simulink model "UZ_EnDat_be4_optimizing_ctrs"  (R2023b)
settings: Solver=FixedStepDiscrete  StartTime=0  StopTime=0.002  RelTol=1e-3
model workspace (MAT data in the model file):
  Select = 0
libraries: hdlsllib x755, simulink x20, simulink_extras x4
(part 5 of 9)

== system UZ_EnDat_be4_optimizing_ctrs/UZ_ENDAT/ManualSerialize/padder/nibblepadding15 ==
  in : Inport
  padding : Subsystem  Commented=through
  padding1 : Subsystem
  padding2 : Subsystem
  padding3 : Subsystem
  out : Outport
  wires:
  in/1 -> padding3/1(in)
  padding2/1(out) -> padding1/1(in)
  padding3/1(out) -> padding2/1(in)
  padding1/1(out) -> padding/1(in)
  padding/1(out) -> out/1

== system UZ_EnDat_be4_optimizing_ctrs/UZ_ENDAT/ManualSerialize/padder/nibblepadding16 ==
  in : Inport
  padding : Subsystem  Commented=through
  padding1 : Subsystem
  padding2 : Subsystem
  padding3 : Subsystem
  out : Outport
  wires:
  in/1 -> padding3/1(in)
  padding2/1(out) -> padding1/1(in)
  padding3/1(out) -> padding2/1(in)
  padding1/1(out) -> padding/1(in)
  padding/1(out) -> out/1

== system UZ_EnDat_be4_optimizing_ctrs/UZ_ENDAT/ManualSerialize/padder/nibblepadding17 ==
  in : Inport
  padding : Subsystem  Commented=through
  padding1 : Subsystem
  padding2 : Subsystem
  padding3 : Subsystem
  out : Outport
  wires:
  in/1 -> padding3/1(in)
  padding2/1(out) -> padding1/1(in)
  padding3/1(out) -> padding2/1(in)
  padding1/1(out) -> padding/1(in)
  padding/1(out) -> out/1

== system UZ_EnDat_be4_optimizing_ctrs/UZ_ENDAT/ManualSerialize/padder/nibblepadding18 ==
  in : Inport
  padding : Subsystem  Commented=through
  padding1 : Subsystem
  padding2 : Subsystem
  padding3 : Subsystem
  out : Outport
  wires:
  in/1 -> padding3/1(in)
  padding2/1(out) -> padding1/1(in)
  padding3/1(out) -> padding2/1(in)
  padding1/1(out) -> padding/1(in)
  padding/1(out) -> out/1

== system UZ_EnDat_be4_optimizing_ctrs/UZ_ENDAT/ManualSerialize/padder/nibblepadding19 ==
  in : Inport
  padding : Subsystem  Commented=through
  padding1 : Subsystem
  padding2 : Subsystem
  padding3 : Subsystem
  out : Outport
  wires:
  in/1 -> padding3/1(in)
  padding2/1(out) -> padding1/1(in)
  padding3/1(out) -> padding2/1(in)
  padding1/1(out) -> padding/1(in)
  padding/1(out) -> out/1

== system UZ_EnDat_be4_optimizing_ctrs/UZ_ENDAT/ManualSerialize/padder/nibblepadding2 ==
  in : Inport
  padding : Subsystem  Commented=through
  padding1 : Subsystem
  padding2 : Subsystem
  padding3 : Subsystem
  out : Outport
  wires:
  in/1 -> padding3/1(in)
  padding2/1(out) -> padding1/1(in)
  padding3/1(out) -> padding2/1(in)
  padding1/1(out) -> padding/1(in)
  padding/1(out) -> out/1

== system UZ_EnDat_be4_optimizing_ctrs/UZ_ENDAT/ManualSerialize/padder/nibblepadding20 ==
  in : Inport
  padding : Subsystem  Commented=through
  padding1 : Subsystem
  padding2 : Subsystem
  padding3 : Subsystem
  out : Outport
  wires:
  in/1 -> padding3/1(in)
  padding2/1(out) -> padding1/1(in)
  padding3/1(out) -> padding2/1(in)
  padding1/1(out) -> padding/1(in)
  padding/1(out) -> out/1

== system UZ_EnDat_be4_optimizing_ctrs/UZ_ENDAT/ManualSerialize/padder/nibblepadding21 ==
  in : Inport
  padding : Subsystem  Commented=through
  padding1 : Subsystem
  padding2 : Subsystem
  padding3 : Subsystem
  out : Outport
  wires:
  in/1 -> padding3/1(in)
  padding2/1(out) -> padding1/1(in)
  padding3/1(out) -> padding2/1(in)
  padding1/1(out) -> padding/1(in)
  padding/1(out) -> out/1

== system UZ_EnDat_be4_optimizing_ctrs/UZ_ENDAT/ManualSerialize/padder/nibblepadding22 ==
  in : Inport
  padding : Subsystem  Commented=through
  padding1 : Subsystem
  padding2 : Subsystem
  padding3 : Subsystem
  out : Outport
  wires:
  in/1 -> padding3/1(in)
  padding2/1(out) -> padding1/1(in)
  padding3/1(out) -> padding2/1(in)
  padding1/1(out) -> padding/1(in)
  padding/1(out) -> out/1

== system UZ_EnDat_be4_optimizing_ctrs/UZ_ENDAT/ManualSerialize/padder/nibblepadding23 ==
  in : Inport
  padding : Subsystem  Commented=through
  padding1 : Subsystem
  padding2 : Subsystem
  padding3 : Subsystem
  out : Outport
  wires:
  in/1 -> padding3/1(in)
  padding2/1(out) -> padding1/1(in)
  padding3/1(out) -> padding2/1(in)
  padding1/1(out) -> padding/1(in)
  padding/1(out) -> out/1

== system UZ_EnDat_be4_optimizing_ctrs/UZ_ENDAT/ManualSerialize/padder/nibblepadding24 ==
  in : Inport
  padding : Subsystem  Commented=through
  padding1 : Subsystem
  padding2 : Subsystem
  padding3 : Subsystem
  out : Outport
  wires:
  in/1 -> padding3/1(in)
  padding2/1(out) -> padding1/1(in)
  padding3/1(out) -> padding2/1(in)
  padding1/1(out) -> padding/1(in)
  padding/1(out) -> out/1

== system UZ_EnDat_be4_optimizing_ctrs/UZ_ENDAT/ManualSerialize/padder/nibblepadding25 ==
  in : Inport
  padding : Subsystem  Commented=through
  padding1 : Subsystem
  padding2 : Subsystem
  padding3 : Subsystem
  out : Outport
  wires:
  in/1 -> padding3/1(in)
  padding2/1(out) -> padding1/1(in)
  padding3/1(out) -> padding2/1(in)
  padding1/1(out) -> padding/1(in)
  padding/1(out) -> out/1

== system UZ_EnDat_be4_optimizing_ctrs/UZ_ENDAT/ManualSerialize/padder/nibblepadding26 ==
  in : Inport
  padding : Subsystem  Commented=through
  padding1 : Subsystem
  padding2 : Subsystem
  padding3 : Subsystem
  out : Outport
  wires:
  in/1 -> padding3/1(in)
  padding2/1(out) -> padding1/1(in)
  padding3/1(out) -> padding2/1(in)
  padding1/1(out) -> padding/1(in)
  padding/1(out) -> out/1

== system UZ_EnDat_be4_optimizing_ctrs/UZ_ENDAT/ManualSerialize/padder/nibblepadding27 ==
  in : Inport
  padding : Subsystem  Commented=through
  padding1 : Subsystem
  padding2 : Subsystem
  padding3 : Subsystem
  out : Outport
  wires:
  in/1 -> padding3/1(in)
  padding2/1(out) -> padding1/1(in)
  padding3/1(out) -> padding2/1(in)
  padding1/1(out) -> padding/1(in)
  padding/1(out) -> out/1

== system UZ_EnDat_be4_optimizing_ctrs/UZ_ENDAT/ManualSerialize/padder/nibblepadding28 ==
  in : Inport
  padding : Subsystem  Commented=through
  padding1 : Subsystem
  padding2 : Subsystem
  padding3 : Subsystem
  out : Outport
  wires:
  in/1 -> padding3/1(in)
  padding2/1(out) -> padding1/1(in)
  padding3/1(out) -> padding2/1(in)
  padding1/1(out) -> padding/1(in)
  padding/1(out) -> out/1

== system UZ_EnDat_be4_optimizing_ctrs/UZ_ENDAT/ManualSerialize/padder/nibblepadding29 ==
  in : Inport
  padding : Subsystem  Commented=through
  padding1 : Subsystem
  padding2 : Subsystem
  padding3 : Subsystem
  out : Outport
  wires:
  in/1 -> padding3/1(in)
  padding2/1(out) -> padding1/1(in)
  padding3/1(out) -> padding2/1(in)
  padding1/1(out) -> padding/1(in)
  padding/1(out) -> out/1

== system UZ_EnDat_be4_optimizing_ctrs/UZ_ENDAT/ManualSerialize/padder/nibblepadding3 ==
  in : Inport
  padding : Subsystem  Commented=through
  padding1 : Subsystem
  padding2 : Subsystem
  padding3 : Subsystem
  out : Outport
  wires:
  in/1 -> padding3/1(in)
  padding2/1(out) -> padding1/1(in)
  padding3/1(out) -> padding2/1(in)
  padding1/1(out) -> padding/1(in)
  padding/1(out) -> out/1

== system UZ_EnDat_be4_optimizing_ctrs/UZ_ENDAT/ManualSerialize/padder/nibblepadding30 ==
  in : Inport
  padding : Subsystem  Commented=through
  padding1 : Subsystem
  padding2 : Subsystem
  padding3 : Subsystem
  out : Outport
  wires:
  in/1 -> padding3/1(in)
  padding2/1(out) -> padding1/1(in)
  padding3/1(out) -> padding2/1(in)
  padding1/1(out) -> padding/1(in)
  padding/1(out) -> out/1

== system UZ_EnDat_be4_optimizing_ctrs/UZ_ENDAT/ManualSerialize/padder/nibblepadding4 ==
  in : Inport
  padding : Subsystem  Commented=through
  padding1 : Subsystem
  padding2 : Subsystem
  padding3 : Subsystem
  out : Outport
  wires:
  in/1 -> padding3/1(in)
  padding2/1(out) -> padding1/1(in)
  padding3/1(out) -> padding2/1(in)
  padding1/1(out) -> padding/1(in)
  padding/1(out) -> out/1

== system UZ_EnDat_be4_optimizing_ctrs/UZ_ENDAT/ManualSerialize/padder/nibblepadding5 ==
  in : Inport
  padding : Subsystem  Commented=through
  padding1 : Subsystem
  padding2 : Subsystem
  padding3 : Subsystem
  out : Outport
  wires:
  in/1 -> padding3/1(in)
  padding2/1(out) -> padding1/1(in)
  padding3/1(out) -> padding2/1(in)
  padding1/1(out) -> padding/1(in)
  padding/1(out) -> out/1

== system UZ_EnDat_be4_optimizing_ctrs/UZ_ENDAT/ManualSerialize/padder/nibblepadding6 ==
  in : Inport
  padding : Subsystem  Commented=through
  padding1 : Subsystem
  padding2 : Subsystem
  padding3 : Subsystem
  out : Outport
  wires:
  in/1 -> padding3/1(in)
  padding2/1(out) -> padding1/1(in)
  padding3/1(out) -> padding2/1(in)
  padding1/1(out) -> padding/1(in)
  padding/1(out) -> out/1

== system UZ_EnDat_be4_optimizing_ctrs/UZ_ENDAT/ManualSerialize/padder/nibblepadding7 ==
  in : Inport
  padding : Subsystem  Commented=through
  padding1 : Subsystem
  padding2 : Subsystem
  padding3 : Subsystem
  out : Outport
  wires:
  in/1 -> padding3/1(in)
  padding2/1(out) -> padding1/1(in)
  padding3/1(out) -> padding2/1(in)
  padding1/1(out) -> padding/1(in)
  padding/1(out) -> out/1

== system UZ_EnDat_be4_optimizing_ctrs/UZ_ENDAT/ManualSerialize/padder/nibblepadding8 ==
  in : Inport
  padding : Subsystem  Commented=through
  padding1 : Subsystem
  padding2 : Subsystem
  padding3 : Subsystem
  out : Outport
  wires:
  in/1 -> padding3/1(in)
  padding2/1(out) -> padding1/1(in)
  padding3/1(out) -> padding2/1(in)
  padding1/1(out) -> padding/1(in)
  padding/1(out) -> out/1

== system UZ_EnDat_be4_optimizing_ctrs/UZ_ENDAT/ManualSerialize/padder/nibblepadding9 ==
  in : Inport
  padding : Subsystem  Commented=through
  padding1 : Subsystem
  padding2 : Subsystem
  padding3 : Subsystem
  out : Outport
  wires:
  in/1 -> padding3/1(in)
  padding2/1(out) -> padding1/1(in)
  padding3/1(out) -> padding2/1(in)
  padding1/1(out) -> padding/1(in)
  padding/1(out) -> out/1

== system UZ_EnDat_be4_optimizing_ctrs/UZ_ENDAT/ManualSerialize1/Storage1/prolonger ==
  in : Inport
  Delay4 : Delay  DelayLength=1
  Logical Operator5 : Logic  Operator=OR  AllPortsSameDT=off  OutDataTypeStr=boolean
  out : Outport
  wires:
  Logical Operator5/1 -> out/1
  in/1 -> Delay4/1, Logical Operator5/1
  Delay4/1 -> Logical Operator5/2

== system UZ_EnDat_be4_optimizing_ctrs/UZ_ENDAT/ManualSerialize1/Storage2/prolonger ==
  in : Inport
  Delay4 : Delay  DelayLength=1
  Logical Operator5 : Logic  Operator=OR  Inputs=3  AllPortsSameDT=off  OutDataTypeStr=boolean
  out : Outport
  wires:
  Logical Operator5/1 -> out/1
  in/1 -> Logical Operator5/3, Delay4/1, Logical Operator5/1
  Delay4/1 -> Logical Operator5/2

== system UZ_EnDat_be4_optimizing_ctrs/UZ_ENDAT/ManualSerialize1/nibblepadding6/padding ==
  in : Inport
  Bit Shift2 : hdlsllib/Logic and Bit Operations/Bit Shift  mode=Shift Right Logical  N=1
  Bit Slice2 : hdlsllib/Logic and Bit Operations/Bit Slice  lidx=0  ridx=0
  Data Type Conversion2 : DataTypeConversion  OutDataTypeStr=boolean  RndMeth=Nearest  SaturateOnIntegerOverflow=off
  Switch2 : Switch  Criteria=u2 > Threshold  SaturateOnIntegerOverflow=off  InputSameDT=off
  out : Outport
  wires:
  in/1 -> Bit Shift2/1, Switch2/1, Bit Slice2/1
  Bit Shift2/1 -> Switch2/3
  Data Type Conversion2/1 -> Switch2/2
  Bit Slice2/1 -> Data Type Conversion2/1
  Switch2/1 -> out/1

== system UZ_EnDat_be4_optimizing_ctrs/UZ_ENDAT/ManualSerialize1/nibblepadding6/padding1 ==
  in : Inport
  Bit Shift2 : hdlsllib/Logic and Bit Operations/Bit Shift  mode=Shift Right Logical  N=1
  Bit Slice2 : hdlsllib/Logic and Bit Operations/Bit Slice  lidx=0  ridx=0
  Data Type Conversion2 : DataTypeConversion  OutDataTypeStr=boolean  RndMeth=Nearest  SaturateOnIntegerOverflow=off
  Switch2 : Switch  Criteria=u2 > Threshold  SaturateOnIntegerOverflow=off  InputSameDT=off
  out : Outport
  wires:
  in/1 -> Bit Shift2/1, Switch2/1, Bit Slice2/1
  Bit Shift2/1 -> Switch2/3
  Data Type Conversion2/1 -> Switch2/2
  Bit Slice2/1 -> Data Type Conversion2/1
  Switch2/1 -> out/1

== system UZ_EnDat_be4_optimizing_ctrs/UZ_ENDAT/ManualSerialize1/nibblepadding6/padding2 ==
  in : Inport
  Bit Shift2 : hdlsllib/Logic and Bit Operations/Bit Shift  mode=Shift Right Logical  N=1
  Bit Slice2 : hdlsllib/Logic and Bit Operations/Bit Slice  lidx=0  ridx=0
  Data Type Conversion2 : DataTypeConversion  OutDataTypeStr=boolean  RndMeth=Nearest  SaturateOnIntegerOverflow=off
  Switch2 : Switch  Criteria=u2 > Threshold  SaturateOnIntegerOverflow=off  InputSameDT=off
  out : Outport
  wires:
  in/1 -> Bit Shift2/1, Switch2/1, Bit Slice2/1
  Bit Shift2/1 -> Switch2/3
  Data Type Conversion2/1 -> Switch2/2
  Bit Slice2/1 -> Data Type Conversion2/1
  Switch2/1 -> out/1

== system UZ_EnDat_be4_optimizing_ctrs/UZ_ENDAT/ManualSerialize1/nibblepadding6/padding3 ==
  in : Inport
  Bit Shift2 : hdlsllib/Logic and Bit Operations/Bit Shift  mode=Shift Right Logical  N=1
  Bit Slice2 : hdlsllib/Logic and Bit Operations/Bit Slice  lidx=0  ridx=0
  Data Type Conversion2 : DataTypeConversion  OutDataTypeStr=boolean  RndMeth=Nearest  SaturateOnIntegerOverflow=off
  Switch2 : Switch  Criteria=u2 > Threshold  SaturateOnIntegerOverflow=off  InputSameDT=off
  out : Outport
  wires:
  in/1 -> Bit Shift2/1, Switch2/1, Bit Slice2/1
  Bit Shift2/1 -> Switch2/3
  Data Type Conversion2/1 -> Switch2/2
  Bit Slice2/1 -> Data Type Conversion2/1
  Switch2/1 -> out/1

== system UZ_EnDat_be4_optimizing_ctrs/UZ_ENDAT/ManualSerialize1/padder/nibblepadding1 ==
  in : Inport
  padding : Subsystem  Commented=through
  padding1 : Subsystem
  padding2 : Subsystem
  padding3 : Subsystem
  out : Outport
  wires:
  in/1 -> padding3/1(in)
  padding2/1(out) -> padding1/1(in)
  padding3/1(out) -> padding2/1(in)
  padding1/1(out) -> padding/1(in)
  padding/1(out) -> out/1

== system UZ_EnDat_be4_optimizing_ctrs/UZ_ENDAT/ManualSerialize1/padder/nibblepadding10 ==
  in : Inport
  padding : Subsystem  Commented=through
  padding1 : Subsystem
  padding2 : Subsystem
  padding3 : Subsystem
  out : Outport
  wires:
  in/1 -> padding3/1(in)
  padding2/1(out) -> padding1/1(in)
  padding3/1(out) -> padding2/1(in)
  padding1/1(out) -> padding/1(in)
  padding/1(out) -> out/1

== system UZ_EnDat_be4_optimizing_ctrs/UZ_ENDAT/ManualSerialize1/padder/nibblepadding11 ==
  in : Inport
  padding : Subsystem  Commented=through
  padding1 : Subsystem
  padding2 : Subsystem
  padding3 : Subsystem
  out : Outport
  wires:
  in/1 -> padding3/1(in)
  padding2/1(out) -> padding1/1(in)
  padding3/1(out) -> padding2/1(in)
  padding1/1(out) -> padding/1(in)
  padding/1(out) -> out/1

== system UZ_EnDat_be4_optimizing_ctrs/UZ_ENDAT/ManualSerialize1/padder/nibblepadding12 ==
  in : Inport
  padding : Subsystem  Commented=through
  padding1 : Subsystem
  padding2 : Subsystem
  padding3 : Subsystem
  out : Outport
  wires:
  in/1 -> padding3/1(in)
  padding2/1(out) -> padding1/1(in)
  padding3/1(out) -> padding2/1(in)
  padding1/1(out) -> padding/1(in)
  padding/1(out) -> out/1

== system UZ_EnDat_be4_optimizing_ctrs/UZ_ENDAT/ManualSerialize1/padder/nibblepadding13 ==
  in : Inport
  padding : Subsystem  Commented=through
  padding1 : Subsystem
  padding2 : Subsystem
  padding3 : Subsystem
  out : Outport
  wires:
  in/1 -> padding3/1(in)
  padding2/1(out) -> padding1/1(in)
  padding3/1(out) -> padding2/1(in)
  padding1/1(out) -> padding/1(in)
  padding/1(out) -> out/1

== system UZ_EnDat_be4_optimizing_ctrs/UZ_ENDAT/ManualSerialize1/padder/nibblepadding14 ==
  in : Inport
  padding : Subsystem  Commented=through
  padding1 : Subsystem
  padding2 : Subsystem
  padding3 : Subsystem
  out : Outport
  wires:
  in/1 -> padding3/1(in)
  padding2/1(out) -> padding1/1(in)
  padding3/1(out) -> padding2/1(in)
  padding1/1(out) -> padding/1(in)
  padding/1(out) -> out/1

== system UZ_EnDat_be4_optimizing_ctrs/UZ_ENDAT/ManualSerialize1/padder/nibblepadding15 ==
  in : Inport
  padding : Subsystem  Commented=through
  padding1 : Subsystem
  padding2 : Subsystem
  padding3 : Subsystem
  out : Outport
  wires:
  in/1 -> padding3/1(in)
  padding2/1(out) -> padding1/1(in)
  padding3/1(out) -> padding2/1(in)
  padding1/1(out) -> padding/1(in)
  padding/1(out) -> out/1

== system UZ_EnDat_be4_optimizing_ctrs/UZ_ENDAT/ManualSerialize1/padder/nibblepadding16 ==
  in : Inport
  padding : Subsystem  Commented=through
  padding1 : Subsystem
  padding2 : Subsystem
  padding3 : Subsystem
  out : Outport
  wires:
  in/1 -> padding3/1(in)
  padding2/1(out) -> padding1/1(in)
  padding3/1(out) -> padding2/1(in)
  padding1/1(out) -> padding/1(in)
  padding/1(out) -> out/1

== system UZ_EnDat_be4_optimizing_ctrs/UZ_ENDAT/ManualSerialize1/padder/nibblepadding17 ==
  in : Inport
  padding : Subsystem  Commented=through
  padding1 : Subsystem
  padding2 : Subsystem
  padding3 : Subsystem
  out : Outport
  wires:
  in/1 -> padding3/1(in)
  padding2/1(out) -> padding1/1(in)
  padding3/1(out) -> padding2/1(in)
  padding1/1(out) -> padding/1(in)
  padding/1(out) -> out/1

== system UZ_EnDat_be4_optimizing_ctrs/UZ_ENDAT/ManualSerialize1/padder/nibblepadding18 ==
  in : Inport
  padding : Subsystem  Commented=through
  padding1 : Subsystem
  padding2 : Subsystem
  padding3 : Subsystem
  out : Outport
  wires:
  in/1 -> padding3/1(in)
  padding2/1(out) -> padding1/1(in)
  padding3/1(out) -> padding2/1(in)
  padding1/1(out) -> padding/1(in)
  padding/1(out) -> out/1

== system UZ_EnDat_be4_optimizing_ctrs/UZ_ENDAT/ManualSerialize1/padder/nibblepadding19 ==
  in : Inport
  padding : Subsystem  Commented=through
  padding1 : Subsystem
  padding2 : Subsystem
  padding3 : Subsystem
  out : Outport
  wires:
  in/1 -> padding3/1(in)
  padding2/1(out) -> padding1/1(in)
  padding3/1(out) -> padding2/1(in)
  padding1/1(out) -> padding/1(in)
  padding/1(out) -> out/1

== system UZ_EnDat_be4_optimizing_ctrs/UZ_ENDAT/ManualSerialize1/padder/nibblepadding2 ==
  in : Inport
  padding : Subsystem  Commented=through
  padding1 : Subsystem
  padding2 : Subsystem
  padding3 : Subsystem
  out : Outport
  wires:
  in/1 -> padding3/1(in)
  padding2/1(out) -> padding1/1(in)
  padding3/1(out) -> padding2/1(in)
  padding1/1(out) -> padding/1(in)
  padding/1(out) -> out/1

== system UZ_EnDat_be4_optimizing_ctrs/UZ_ENDAT/ManualSerialize1/padder/nibblepadding20 ==
  in : Inport
  padding : Subsystem  Commented=through
  padding1 : Subsystem
  padding2 : Subsystem
  padding3 : Subsystem
  out : Outport
  wires:
  in/1 -> padding3/1(in)
  padding2/1(out) -> padding1/1(in)
  padding3/1(out) -> padding2/1(in)
  padding1/1(out) -> padding/1(in)
  padding/1(out) -> out/1

== system UZ_EnDat_be4_optimizing_ctrs/UZ_ENDAT/ManualSerialize1/padder/nibblepadding21 ==
  in : Inport
  padding : Subsystem  Commented=through
  padding1 : Subsystem
  padding2 : Subsystem
  padding3 : Subsystem
  out : Outport
  wires:
  in/1 -> padding3/1(in)
  padding2/1(out) -> padding1/1(in)
  padding3/1(out) -> padding2/1(in)
  padding1/1(out) -> padding/1(in)
  padding/1(out) -> out/1

== system UZ_EnDat_be4_optimizing_ctrs/UZ_ENDAT/ManualSerialize1/padder/nibblepadding22 ==
  in : Inport
  padding : Subsystem  Commented=through
  padding1 : Subsystem
  padding2 : Subsystem
  padding3 : Subsystem
  out : Outport
  wires:
  in/1 -> padding3/1(in)
  padding2/1(out) -> padding1/1(in)
  padding3/1(out) -> padding2/1(in)
  padding1/1(out) -> padding/1(in)
  padding/1(out) -> out/1

== system UZ_EnDat_be4_optimizing_ctrs/UZ_ENDAT/ManualSerialize1/padder/nibblepadding23 ==
  in : Inport
  padding : Subsystem  Commented=through
  padding1 : Subsystem
  padding2 : Subsystem
  padding3 : Subsystem
  out : Outport
  wires:
  in/1 -> padding3/1(in)
  padding2/1(out) -> padding1/1(in)
  padding3/1(out) -> padding2/1(in)
  padding1/1(out) -> padding/1(in)
  padding/1(out) -> out/1

== system UZ_EnDat_be4_optimizing_ctrs/UZ_ENDAT/ManualSerialize1/padder/nibblepadding24 ==
  in : Inport
  padding : Subsystem  Commented=through
  padding1 : Subsystem
  padding2 : Subsystem
  padding3 : Subsystem
  out : Outport
  wires:
  in/1 -> padding3/1(in)
  padding2/1(out) -> padding1/1(in)
  padding3/1(out) -> padding2/1(in)
  padding1/1(out) -> padding/1(in)
  padding/1(out) -> out/1

== system UZ_EnDat_be4_optimizing_ctrs/UZ_ENDAT/ManualSerialize1/padder/nibblepadding25 ==
  in : Inport
  padding : Subsystem  Commented=through
  padding1 : Subsystem
  padding2 : Subsystem
  padding3 : Subsystem
  out : Outport
  wires:
  in/1 -> padding3/1(in)
  padding2/1(out) -> padding1/1(in)
  padding3/1(out) -> padding2/1(in)
  padding1/1(out) -> padding/1(in)
  padding/1(out) -> out/1

== system UZ_EnDat_be4_optimizing_ctrs/UZ_ENDAT/ManualSerialize1/padder/nibblepadding26 ==
  in : Inport
  padding : Subsystem  Commented=through
  padding1 : Subsystem
  padding2 : Subsystem
  padding3 : Subsystem
  out : Outport
  wires:
  in/1 -> padding3/1(in)
  padding2/1(out) -> padding1/1(in)
  padding3/1(out) -> padding2/1(in)
  padding1/1(out) -> padding/1(in)
  padding/1(out) -> out/1

== system UZ_EnDat_be4_optimizing_ctrs/UZ_ENDAT/ManualSerialize1/padder/nibblepadding27 ==
  in : Inport
  padding : Subsystem  Commented=through
  padding1 : Subsystem
  padding2 : Subsystem
  padding3 : Subsystem
  out : Outport
  wires:
  in/1 -> padding3/1(in)
  padding2/1(out) -> padding1/1(in)
  padding3/1(out) -> padding2/1(in)
  padding1/1(out) -> padding/1(in)
  padding/1(out) -> out/1

== system UZ_EnDat_be4_optimizing_ctrs/UZ_ENDAT/ManualSerialize1/padder/nibblepadding28 ==
  in : Inport
  padding : Subsystem  Commented=through
  padding1 : Subsystem
  padding2 : Subsystem
  padding3 : Subsystem
  out : Outport
  wires:
  in/1 -> padding3/1(in)
  padding2/1(out) -> padding1/1(in)
  padding3/1(out) -> padding2/1(in)
  padding1/1(out) -> padding/1(in)
  padding/1(out) -> out/1

== system UZ_EnDat_be4_optimizing_ctrs/UZ_ENDAT/ManualSerialize1/padder/nibblepadding29 ==
  in : Inport
  padding : Subsystem  Commented=through
  padding1 : Subsystem
  padding2 : Subsystem
  padding3 : Subsystem
  out : Outport
  wires:
  in/1 -> padding3/1(in)
  padding2/1(out) -> padding1/1(in)
  padding3/1(out) -> padding2/1(in)
  padding1/1(out) -> padding/1(in)
  padding/1(out) -> out/1

== system UZ_EnDat_be4_optimizing_ctrs/UZ_ENDAT/ManualSerialize1/padder/nibblepadding3 ==
  in : Inport
  padding : Subsystem  Commented=through
  padding1 : Subsystem
  padding2 : Subsystem
  padding3 : Subsystem
  out : Outport
  wires:
  in/1 -> padding3/1(in)
  padding2/1(out) -> padding1/1(in)
  padding3/1(out) -> padding2/1(in)
  padding1/1(out) -> padding/1(in)
  padding/1(out) -> out/1

== system UZ_EnDat_be4_optimizing_ctrs/UZ_ENDAT/ManualSerialize1/padder/nibblepadding4 ==
  in : Inport
  padding : Subsystem  Commented=through
  padding1 : Subsystem
  padding2 : Subsystem
  padding3 : Subsystem
  out : Outport
  wires:
  in/1 -> padding3/1(in)
  padding2/1(out) -> padding1/1(in)
  padding3/1(out) -> padding2/1(in)
  padding1/1(out) -> padding/1(in)
  padding/1(out) -> out/1

== system UZ_EnDat_be4_optimizing_ctrs/UZ_ENDAT/ManualSerialize1/padder/nibblepadding5 ==
  in : Inport
  padding : Subsystem  Commented=through
  padding1 : Subsystem
  padding2 : Subsystem
  padding3 : Subsystem
  out : Outport
  wires:
  in/1 -> padding3/1(in)
  padding2/1(out) -> padding1/1(in)
  padding3/1(out) -> padding2/1(in)
  padding1/1(out) -> padding/1(in)
  padding/1(out) -> out/1

== system UZ_EnDat_be4_optimizing_ctrs/UZ_ENDAT/ManualSerialize1/padder/nibblepadding6 ==
  in : Inport
  padding : Subsystem  Commented=through
  padding1 : Subsystem
  padding2 : Subsystem
  padding3 : Subsystem
  out : Outport
  wires:
  in/1 -> padding3/1(in)
  padding2/1(out) -> padding1/1(in)
  padding3/1(out) -> padding2/1(in)
  padding1/1(out) -> padding/1(in)
  padding/1(out) -> out/1

== system UZ_EnDat_be4_optimizing_ctrs/UZ_ENDAT/ManualSerialize1/padder/nibblepadding7 ==
  in : Inport
  padding : Subsystem  Commented=through
  padding1 : Subsystem
  padding2 : Subsystem
  padding3 : Subsystem
  out : Outport
  wires:
  in/1 -> padding3/1(in)
  padding2/1(out) -> padding1/1(in)
  padding3/1(out) -> padding2/1(in)
  padding1/1(out) -> padding/1(in)
  padding/1(out) -> out/1

== system UZ_EnDat_be4_optimizing_ctrs/UZ_ENDAT/ManualSerialize1/padder/nibblepadding8 ==
  in : Inport
  padding : Subsystem  Commented=through
  padding1 : Subsystem
  padding2 : Subsystem
  padding3 : Subsystem
  out : Outport
  wires:
  in/1 -> padding3/1(in)
  padding2/1(out) -> padding1/1(in)
  padding3/1(out) -> padding2/1(in)
  padding1/1(out) -> padding/1(in)
  padding/1(out) -> out/1

== system UZ_EnDat_be4_optimizing_ctrs/UZ_ENDAT/ManualSerialize1/padder/nibblepadding9 ==
  in : Inport
  padding : Subsystem  Commented=through
  padding1 : Subsystem
  padding2 : Subsystem
  padding3 : Subsystem
  out : Outport
  wires:
  in/1 -> padding3/1(in)
  padding2/1(out) -> padding1/1(in)
  padding3/1(out) -> padding2/1(in)
  padding1/1(out) -> padding/1(in)
  padding/1(out) -> out/1

== system UZ_EnDat_be4_optimizing_ctrs/UZ_ENDAT/RESPONSESLICER3X/19BITSLICER/responseslicer ==
  DATA : Inport  OutDataTypeStr=uint64
  Bit Slice1 : hdlsllib/Logic and Bit Operations/Bit Slice  lidx=1  ridx=1
  Bit Slice3 : hdlsllib/Logic and Bit Operations/Bit Slice  lidx=25  ridx=21
  Bit Slice4 : hdlsllib/Logic and Bit Operations/Bit Slice  lidx=20  ridx=2
  Data Type Conversion1 : DataTypeConversion  OutDataTypeStr=boolean  SaturateOnIntegerOverflow=off  RndMeth=Floor
  Data Type Conversion3 : DataTypeConversion  OutDataTypeStr=uint8  SaturateOnIntegerOverflow=off  RndMeth=Floor
  Data Type Conversion4 : DataTypeConversion  OutDataTypeStr=uint32  SaturateOnIntegerOverflow=off  RndMeth=Floor
  Terminator : Terminator
  CRC : Outport  OutDataTypeStr=uint8
  payload : Outport  Port=2  OutDataTypeStr=uint32
  error : Outport  Port=3  OutDataTypeStr=boolean
  wires:
  DATA/1 -> Terminator/1, Bit Slice1/1, Bit Slice4/1, Bit Slice3/1
  Bit Slice3/1 -> Data Type Conversion3/1
  Bit Slice4/1 -> Data Type Conversion4/1
  Data Type Conversion3/1 -> CRC/1
  Data Type Conversion4/1 -> payload/1
  Bit Slice1/1 -> Data Type Conversion1/1
  Data Type Conversion1/1 -> error/1

== system UZ_EnDat_be4_optimizing_ctrs/UZ_ENDAT/RESPONSESLICER3X/19BITSLICER/responseslicer1 ==
  DATA : Inport  OutDataTypeStr=uint64
  Bit Slice1 : hdlsllib/Logic and Bit Operations/Bit Slice  lidx=1  ridx=1
  Bit Slice3 : hdlsllib/Logic and Bit Operations/Bit Slice  lidx=25  ridx=21
  Bit Slice4 : hdlsllib/Logic and Bit Operations/Bit Slice  lidx=20  ridx=2
  Data Type Conversion1 : DataTypeConversion  OutDataTypeStr=boolean  SaturateOnIntegerOverflow=off  RndMeth=Floor
  Data Type Conversion3 : DataTypeConversion  OutDataTypeStr=uint8  SaturateOnIntegerOverflow=off  RndMeth=Floor
  Data Type Conversion4 : DataTypeConversion  OutDataTypeStr=uint32  SaturateOnIntegerOverflow=off  RndMeth=Floor
  Terminator : Terminator
  CRC : Outport  OutDataTypeStr=uint8
  payload : Outport  Port=2  OutDataTypeStr=uint32
  error : Outport  Port=3  OutDataTypeStr=boolean
  wires:
  DATA/1 -> Terminator/1, Bit Slice1/1, Bit Slice4/1, Bit Slice3/1
  Bit Slice3/1 -> Data Type Conversion3/1
  Bit Slice4/1 -> Data Type Conversion4/1
  Data Type Conversion3/1 -> CRC/1
  Data Type Conversion4/1 -> payload/1
  Bit Slice1/1 -> Data Type Conversion1/1
  Data Type Conversion1/1 -> error/1

== system UZ_EnDat_be4_optimizing_ctrs/UZ_ENDAT/RESPONSESLICER3X/19BITSLICER/responseslicer2 ==
  DATA : Inport  OutDataTypeStr=uint64
  Bit Slice1 : hdlsllib/Logic and Bit Operations/Bit Slice  lidx=1  ridx=1
  Bit Slice3 : hdlsllib/Logic and Bit Operations/Bit Slice  lidx=25  ridx=21
  Bit Slice4 : hdlsllib/Logic and Bit Operations/Bit Slice  lidx=20  ridx=2
  Data Type Conversion1 : DataTypeConversion  OutDataTypeStr=boolean  SaturateOnIntegerOverflow=off  RndMeth=Floor
  Data Type Conversion3 : DataTypeConversion  OutDataTypeStr=uint8  SaturateOnIntegerOverflow=off  RndMeth=Floor
  Data Type Conversion4 : DataTypeConversion  OutDataTypeStr=uint32  SaturateOnIntegerOverflow=off  RndMeth=Floor
  Terminator : Terminator
  CRC : Outport  OutDataTypeStr=uint8
  payload : Outport  Port=2  OutDataTypeStr=uint32
  error : Outport  Port=3  OutDataTypeStr=boolean
  wires:
  DATA/1 -> Terminator/1, Bit Slice1/1, Bit Slice4/1, Bit Slice3/1
  Bit Slice3/1 -> Data Type Conversion3/1
  Bit Slice4/1 -> Data Type Conversion4/1
  Data Type Conversion3/1 -> CRC/1
  Data Type Conversion4/1 -> payload/1
  Bit Slice1/1 -> Data Type Conversion1/1
  Data Type Conversion1/1 -> error/1

== system UZ_EnDat_be4_optimizing_ctrs/UZ_ENDAT/RESPONSESLICER3X/21BITSLICER/responseslicer ==
  DATA : Inport  OutDataTypeStr=uint64
  Bit Slice1 : hdlsllib/Logic and Bit Operations/Bit Slice  lidx=1  ridx=1
  Bit Slice3 : hdlsllib/Logic and Bit Operations/Bit Slice  lidx=27  ridx=23
  Bit Slice4 : hdlsllib/Logic and Bit Operations/Bit Slice  lidx=22  ridx=2
  Data Type Conversion1 : DataTypeConversion  OutDataTypeStr=boolean  SaturateOnIntegerOverflow=off  RndMeth=Floor
  Data Type Conversion3 : DataTypeConversion  OutDataTypeStr=uint8  SaturateOnIntegerOverflow=off  RndMeth=Floor
  Data Type Conversion4 : DataTypeConversion  OutDataTypeStr=uint32  SaturateOnIntegerOverflow=off  RndMeth=Floor
  Terminator : Terminator
  CRC : Outport  OutDataTypeStr=uint8
  payload : Outport  Port=2  OutDataTypeStr=uint32
  error : Outport  Port=3  OutDataTypeStr=boolean
  wires:
  DATA/1 -> Terminator/1, Bit Slice1/1, Bit Slice4/1, Bit Slice3/1
  Bit Slice3/1 -> Data Type Conversion3/1
  Bit Slice4/1 -> Data Type Conversion4/1
  Data Type Conversion3/1 -> CRC/1
  Data Type Conversion4/1 -> payload/1
  Bit Slice1/1 -> Data Type Conversion1/1
  Data Type Conversion1/1 -> error/1

== system UZ_EnDat_be4_optimizing_ctrs/UZ_ENDAT/RESPONSESLICER3X/21BITSLICER/responseslicer3 ==
  DATA : Inport  OutDataTypeStr=uint64
  Bit Slice1 : hdlsllib/Logic and Bit Operations/Bit Slice  lidx=1  ridx=1
  Bit Slice3 : hdlsllib/Logic and Bit Operations/Bit Slice  lidx=27  ridx=23
  Bit Slice4 : hdlsllib/Logic and Bit Operations/Bit Slice  lidx=22  ridx=2
  Data Type Conversion1 : DataTypeConversion  OutDataTypeStr=boolean  SaturateOnIntegerOverflow=off  RndMeth=Floor
  Data Type Conversion3 : DataTypeConversion  OutDataTypeStr=uint8  SaturateOnIntegerOverflow=off  RndMeth=Floor
  Data Type Conversion4 : DataTypeConversion  OutDataTypeStr=uint32  SaturateOnIntegerOverflow=off  RndMeth=Floor
  Terminator : Terminator
  CRC : Outport  OutDataTypeStr=uint8
  payload : Outport  Port=2  OutDataTypeStr=uint32
  error : Outport  Port=3  OutDataTypeStr=boolean
  wires:
  DATA/1 -> Terminator/1, Bit Slice1/1, Bit Slice4/1, Bit Slice3/1
  Bit Slice3/1 -> Data Type Conversion3/1
  Bit Slice4/1 -> Data Type Conversion4/1
  Data Type Conversion3/1 -> CRC/1
  Data Type Conversion4/1 -> payload/1
  Bit Slice1/1 -> Data Type Conversion1/1
  Data Type Conversion1/1 -> error/1

== system UZ_EnDat_be4_optimizing_ctrs/UZ_ENDAT/RESPONSESLICER3X/21BITSLICER/responseslicer4 ==
  DATA : Inport  OutDataTypeStr=uint64
  Bit Slice1 : hdlsllib/Logic and Bit Operations/Bit Slice  lidx=1  ridx=1
  Bit Slice3 : hdlsllib/Logic and Bit Operations/Bit Slice  lidx=27  ridx=23
  Bit Slice4 : hdlsllib/Logic and Bit Operations/Bit Slice  lidx=22  ridx=2
  Data Type Conversion1 : DataTypeConversion  OutDataTypeStr=boolean  SaturateOnIntegerOverflow=off  RndMeth=Floor
  Data Type Conversion3 : DataTypeConversion  OutDataTypeStr=uint8  SaturateOnIntegerOverflow=off  RndMeth=Floor
  Data Type Conversion4 : DataTypeConversion  OutDataTypeStr=uint32  SaturateOnIntegerOverflow=off  RndMeth=Floor
  Terminator : Terminator
  CRC : Outport  OutDataTypeStr=uint8
  payload : Outport  Port=2  OutDataTypeStr=uint32
  error : Outport  Port=3  OutDataTypeStr=boolean
  wires:
  DATA/1 -> Terminator/1, Bit Slice1/1, Bit Slice4/1, Bit Slice3/1
  Bit Slice3/1 -> Data Type Conversion3/1
  Bit Slice4/1 -> Data Type Conversion4/1
  Data Type Conversion3/1 -> CRC/1
  Data Type Conversion4/1 -> payload/1
  Bit Slice1/1 -> Data Type Conversion1/1
  Data Type Conversion1/1 -> error/1

== system UZ_EnDat_be4_optimizing_ctrs/UZ_ENDAT/RESPONSESLICER3X/23BITSLICER/responseslicer ==
  DATA : Inport  OutDataTypeStr=uint64
  Bit Slice1 : hdlsllib/Logic and Bit Operations/Bit Slice  lidx=1  ridx=1
  Bit Slice3 : hdlsllib/Logic and Bit Operations/Bit Slice  lidx=29  ridx=25
  Bit Slice4 : hdlsllib/Logic and Bit Operations/Bit Slice  lidx=24  ridx=2
  Data Type Conversion1 : DataTypeConversion  OutDataTypeStr=boolean  SaturateOnIntegerOverflow=off  RndMeth=Floor
  Data Type Conversion3 : DataTypeConversion  OutDataTypeStr=uint8  SaturateOnIntegerOverflow=off  RndMeth=Floor
  Data Type Conversion4 : DataTypeConversion  OutDataTypeStr=uint32  SaturateOnIntegerOverflow=off  RndMeth=Floor
  Terminator : Terminator
  CRC : Outport  OutDataTypeStr=uint8
  payload : Outport  Port=2  OutDataTypeStr=uint32
  error : Outport  Port=3  OutDataTypeStr=boolean
  wires:
  DATA/1 -> Terminator/1, Bit Slice1/1, Bit Slice4/1, Bit Slice3/1
  Bit Slice3/1 -> Data Type Conversion3/1
  Bit Slice4/1 -> Data Type Conversion4/1
  Data Type Conversion3/1 -> CRC/1
  Data Type Conversion4/1 -> payload/1
  Bit Slice1/1 -> Data Type Conversion1/1
  Data Type Conversion1/1 -> error/1

== system UZ_EnDat_be4_optimizing_ctrs/UZ_ENDAT/RESPONSESLICER3X/23BITSLICER/responseslicer1 ==
  DATA : Inport  OutDataTypeStr=uint64
  Bit Slice1 : hdlsllib/Logic and Bit Operations/Bit Slice  lidx=1  ridx=1
  Bit Slice3 : hdlsllib/Logic and Bit Operations/Bit Slice  lidx=29  ridx=25
  Bit Slice4 : hdlsllib/Logic and Bit Operations/Bit Slice  lidx=24  ridx=2
  Data Type Conversion1 : DataTypeConversion  OutDataTypeStr=boolean  SaturateOnIntegerOverflow=off  RndMeth=Floor
  Data Type Conversion3 : DataTypeConversion  OutDataTypeStr=uint8  SaturateOnIntegerOverflow=off  RndMeth=Floor
  Data Type Conversion4 : DataTypeConversion  OutDataTypeStr=uint32  SaturateOnIntegerOverflow=off  RndMeth=Floor
  Terminator : Terminator
  CRC : Outport  OutDataTypeStr=uint8
  payload : Outport  Port=2  OutDataTypeStr=uint32
  error : Outport  Port=3  OutDataTypeStr=boolean
  wires:
  DATA/1 -> Terminator/1, Bit Slice1/1, Bit Slice4/1, Bit Slice3/1
  Bit Slice3/1 -> Data Type Conversion3/1
  Bit Slice4/1 -> Data Type Conversion4/1
  Data Type Conversion3/1 -> CRC/1
  Data Type Conversion4/1 -> payload/1
  Bit Slice1/1 -> Data Type Conversion1/1
  Data Type Conversion1/1 -> error/1

== system UZ_EnDat_be4_optimizing_ctrs/UZ_ENDAT/RESPONSESLICER3X/23BITSLICER/responseslicer2 ==
  DATA : Inport  OutDataTypeStr=uint64
  Bit Slice1 : hdlsllib/Logic and Bit Operations/Bit Slice  lidx=1  ridx=1
  Bit Slice3 : hdlsllib/Logic and Bit Operations/Bit Slice  lidx=29  ridx=25
  Bit Slice4 : hdlsllib/Logic and Bit Operations/Bit Slice  lidx=24  ridx=2
  Data Type Conversion1 : DataTypeConversion  OutDataTypeStr=boolean  SaturateOnIntegerOverflow=off  RndMeth=Floor
  Data Type Conversion3 : DataTypeConversion  OutDataTypeStr=uint8  SaturateOnIntegerOverflow=off  RndMeth=Floor
  Data Type Conversion4 : DataTypeConversion  OutDataTypeStr=uint32  SaturateOnIntegerOverflow=off  RndMeth=Floor
  Terminator : Terminator
  CRC : Outport  OutDataTypeStr=uint8
  payload : Outport  Port=2  OutDataTypeStr=uint32
  error : Outport  Port=3  OutDataTypeStr=boolean
  wires:
  DATA/1 -> Terminator/1, Bit Slice1/1, Bit Slice4/1, Bit Slice3/1
  Bit Slice3/1 -> Data Type Conversion3/1
  Bit Slice4/1 -> Data Type Conversion4/1
  Data Type Conversion3/1 -> CRC/1
  Data Type Conversion4/1 -> payload/1
  Bit Slice1/1 -> Data Type Conversion1/1
  Data Type Conversion1/1 -> error/1

== system UZ_EnDat_be4_optimizing_ctrs/UZ_ENDAT/RESPONSESLICER3X/25BITSLICER/responseslicer ==
  DATA : Inport  OutDataTypeStr=uint64
  Bit Slice1 : hdlsllib/Logic and Bit Operations/Bit Slice  lidx=1  ridx=1
  Bit Slice3 : hdlsllib/Logic and Bit Operations/Bit Slice  lidx=31  ridx=27
  Bit Slice4 : hdlsllib/Logic and Bit Operations/Bit Slice  lidx=26  ridx=2
  Data Type Conversion1 : DataTypeConversion  OutDataTypeStr=boolean  SaturateOnIntegerOverflow=off  RndMeth=Floor
  Data Type Conversion3 : DataTypeConversion  OutDataTypeStr=uint8  SaturateOnIntegerOverflow=off  RndMeth=Floor
  Data Type Conversion4 : DataTypeConversion  OutDataTypeStr=uint32  SaturateOnIntegerOverflow=off  RndMeth=Floor
  Terminator : Terminator
  CRC : Outport  OutDataTypeStr=uint8
  payload : Outport  Port=2  OutDataTypeStr=uint32
  error : Outport  Port=3  OutDataTypeStr=boolean
  wires:
  DATA/1 -> Terminator/1, Bit Slice1/1, Bit Slice4/1, Bit Slice3/1
  Bit Slice3/1 -> Data Type Conversion3/1
  Bit Slice4/1 -> Data Type Conversion4/1
  Data Type Conversion3/1 -> CRC/1
  Data Type Conversion4/1 -> payload/1
  Bit Slice1/1 -> Data Type Conversion1/1
  Data Type Conversion1/1 -> error/1

== system UZ_EnDat_be4_optimizing_ctrs/UZ_ENDAT/RESPONSESLICER3X/25BITSLICER/responseslicer1 ==
  DATA : Inport  OutDataTypeStr=uint64
  Bit Slice1 : hdlsllib/Logic and Bit Operations/Bit Slice  lidx=1  ridx=1
  Bit Slice3 : hdlsllib/Logic and Bit Operations/Bit Slice  lidx=31  ridx=27
  Bit Slice4 : hdlsllib/Logic and Bit Operations/Bit Slice  lidx=26  ridx=2
  Data Type Conversion1 : DataTypeConversion  OutDataTypeStr=boolean  SaturateOnIntegerOverflow=off  RndMeth=Floor
  Data Type Conversion3 : DataTypeConversion  OutDataTypeStr=uint8  SaturateOnIntegerOverflow=off  RndMeth=Floor
  Data Type Conversion4 : DataTypeConversion  OutDataTypeStr=uint32  SaturateOnIntegerOverflow=off  RndMeth=Floor
  Terminator : Terminator
  CRC : Outport  OutDataTypeStr=uint8
  payload : Outport  Port=2  OutDataTypeStr=uint32
  error : Outport  Port=3  OutDataTypeStr=boolean
  wires:
  DATA/1 -> Terminator/1, Bit Slice1/1, Bit Slice4/1, Bit Slice3/1
  Bit Slice3/1 -> Data Type Conversion3/1
  Bit Slice4/1 -> Data Type Conversion4/1
  Data Type Conversion3/1 -> CRC/1
  Data Type Conversion4/1 -> payload/1
  Bit Slice1/1 -> Data Type Conversion1/1
  Data Type Conversion1/1 -> error/1

== system UZ_EnDat_be4_optimizing_ctrs/UZ_ENDAT/RESPONSESLICER3X/25BITSLICER/responseslicer2 ==
  DATA : Inport  OutDataTypeStr=uint64
  Bit Slice1 : hdlsllib/Logic and Bit Operations/Bit Slice  lidx=1  ridx=1
  Bit Slice3 : hdlsllib/Logic and Bit Operations/Bit Slice  lidx=31  ridx=27
  Bit Slice4 : hdlsllib/Logic and Bit Operations/Bit Slice  lidx=26  ridx=2
  Data Type Conversion1 : DataTypeConversion  OutDataTypeStr=boolean  SaturateOnIntegerOverflow=off  RndMeth=Floor
  Data Type Conversion3 : DataTypeConversion  OutDataTypeStr=uint8  SaturateOnIntegerOverflow=off  RndMeth=Floor
  Data Type Conversion4 : DataTypeConversion  OutDataTypeStr=uint32  SaturateOnIntegerOverflow=off  RndMeth=Floor
  Terminator : Terminator
  CRC : Outport  OutDataTypeStr=uint8
  payload : Outport  Port=2  OutDataTypeStr=uint32
  error : Outport  Port=3  OutDataTypeStr=boolean
  wires:
  DATA/1 -> Terminator/1, Bit Slice1/1, Bit Slice4/1, Bit Slice3/1
  Bit Slice3/1 -> Data Type Conversion3/1
  Bit Slice4/1 -> Data Type Conversion4/1
  Data Type Conversion3/1 -> CRC/1
  Data Type Conversion4/1 -> payload/1
  Bit Slice1/1 -> Data Type Conversion1/1
  Data Type Conversion1/1 -> error/1

== system UZ_EnDat_be4_optimizing_ctrs/UZ_ENDAT/RESPONSESLICER3X/27BITSLICER/responseslicer ==
  DATA : Inport  OutDataTypeStr=uint64
  Bit Slice1 : hdlsllib/Logic and Bit Operations/Bit Slice  lidx=1  ridx=1
  Bit Slice3 : hdlsllib/Logic and Bit Operations/Bit Slice  lidx=33  ridx=29
  Bit Slice4 : hdlsllib/Logic and Bit Operations/Bit Slice  lidx=28  ridx=2
  Data Type Conversion1 : DataTypeConversion  OutDataTypeStr=boolean  SaturateOnIntegerOverflow=off  RndMeth=Floor
  Data Type Conversion3 : DataTypeConversion  OutDataTypeStr=uint8  SaturateOnIntegerOverflow=off  RndMeth=Floor
  Data Type Conversion4 : DataTypeConversion  OutDataTypeStr=uint32  SaturateOnIntegerOverflow=off  RndMeth=Floor
  Terminator : Terminator
  CRC : Outport  OutDataTypeStr=uint8
  payload : Outport  Port=2  OutDataTypeStr=uint32
  error : Outport  Port=3  OutDataTypeStr=boolean
  wires:
  DATA/1 -> Terminator/1, Bit Slice1/1, Bit Slice4/1, Bit Slice3/1
  Bit Slice3/1 -> Data Type Conversion3/1
  Bit Slice4/1 -> Data Type Conversion4/1
  Data Type Conversion3/1 -> CRC/1
  Data Type Conversion4/1 -> payload/1
  Bit Slice1/1 -> Data Type Conversion1/1
  Data Type Conversion1/1 -> error/1

== system UZ_EnDat_be4_optimizing_ctrs/UZ_ENDAT/RESPONSESLICER3X/27BITSLICER/responseslicer1 ==
  DATA : Inport  OutDataTypeStr=uint64
  Bit Slice1 : hdlsllib/Logic and Bit Operations/Bit Slice  lidx=1  ridx=1
  Bit Slice3 : hdlsllib/Logic and Bit Operations/Bit Slice  lidx=33  ridx=29
  Bit Slice4 : hdlsllib/Logic and Bit Operations/Bit Slice  lidx=28  ridx=2
  Data Type Conversion1 : DataTypeConversion  OutDataTypeStr=boolean  SaturateOnIntegerOverflow=off  RndMeth=Floor
  Data Type Conversion3 : DataTypeConversion  OutDataTypeStr=uint8  SaturateOnIntegerOverflow=off  RndMeth=Floor
  Data Type Conversion4 : DataTypeConversion  OutDataTypeStr=uint32  SaturateOnIntegerOverflow=off  RndMeth=Floor
  Terminator : Terminator
  CRC : Outport  OutDataTypeStr=uint8
  payload : Outport  Port=2  OutDataTypeStr=uint32
  error : Outport  Port=3  OutDataTypeStr=boolean
  wires:
  DATA/1 -> Terminator/1, Bit Slice1/1, Bit Slice4/1, Bit Slice3/1
  Bit Slice3/1 -> Data Type Conversion3/1
  Bit Slice4/1 -> Data Type Conversion4/1
  Data Type Conversion3/1 -> CRC/1
  Data Type Conversion4/1 -> payload/1
  Bit Slice1/1 -> Data Type Conversion1/1
  Data Type Conversion1/1 -> error/1

== system UZ_EnDat_be4_optimizing_ctrs/UZ_ENDAT/RESPONSESLICER3X/27BITSLICER/responseslicer2 ==
  DATA : Inport  OutDataTypeStr=uint64
  Bit Slice1 : hdlsllib/Logic and Bit Operations/Bit Slice  lidx=1  ridx=1
  Bit Slice3 : hdlsllib/Logic and Bit Operations/Bit Slice  lidx=33  ridx=29
  Bit Slice4 : hdlsllib/Logic and Bit Operations/Bit Slice  lidx=28  ridx=2
  Data Type Conversion1 : DataTypeConversion  OutDataTypeStr=boolean  SaturateOnIntegerOverflow=off  RndMeth=Floor
  Data Type Conversion3 : DataTypeConversion  OutDataTypeStr=uint8  SaturateOnIntegerOverflow=off  RndMeth=Floor
  Data Type Conversion4 : DataTypeConversion  OutDataTypeStr=uint32  SaturateOnIntegerOverflow=off  RndMeth=Floor
  Terminator : Terminator
  CRC : Outport  OutDataTypeStr=uint8
  payload : Outport  Port=2  OutDataTypeStr=uint32
  error : Outport  Port=3  OutDataTypeStr=boolean
  wires:
  DATA/1 -> Terminator/1, Bit Slice1/1, Bit Slice4/1, Bit Slice3/1
  Bit Slice3/1 -> Data Type Conversion3/1
  Bit Slice4/1 -> Data Type Conversion4/1
  Data Type Conversion3/1 -> CRC/1
  Data Type Conversion4/1 -> payload/1
  Bit Slice1/1 -> Data Type Conversion1/1
  Data Type Conversion1/1 -> error/1

== system UZ_EnDat_be4_optimizing_ctrs/UZ_ENDAT/Subsystem2/ManualDeserializere/WORDTOBOOL ==
  DATAIN : Inport
  Trigger : TriggerPort  TriggerType=falling  VariantControl=(inherit)  OutputDataType=int8  InitialTriggerSignalState=positive
  Data Type Conversion{,1..15} (16 alike) : DataTypeConversion  OutDataTypeStr=boolean  SaturateOnIntegerOverflow=off  RndMeth=Floor
  Demux : Demux  Outputs=16
  Word to Bits : hdlsllib/Logic and Bit Operations/Word to Bits  maxWordLength=16
  DATAOUT0 : Outport  InitialOutput=0
  DATAOUT1 : Outport  Port=2  InitialOutput=0
  DATAOUT2 : Outport  Port=3  InitialOutput=0
  DATAOUT3 : Outport  Port=4  InitialOutput=0
  DATAOUT4 : Outport  Port=5  InitialOutput=0
  DATAOUT5 : Outport  Port=6  InitialOutput=0
  DATAOUT6 : Outport  Port=7  InitialOutput=0
  DATAOUT7 : Outport  Port=8  InitialOutput=0
  DATAOUT8 : Outport  Port=9  InitialOutput=0
  DATAOUT9 : Outport  Port=10  InitialOutput=0
  DATAOUT10 : Outport  Port=11  InitialOutput=0
  DATAOUT11 : Outport  Port=12  InitialOutput=0
  DATAOUT12 : Outport  Port=13  InitialOutput=0
  DATAOUT13 : Outport  Port=14  InitialOutput=0
  DATAOUT14 : Outport  Port=15  InitialOutput=0
  DATAOUT15 : Outport  Port=16  InitialOutput=0
  wires:
  Demux/1 -> Data Type Conversion/1
  Demux/2 -> Data Type Conversion1/1
  Demux/4 -> Data Type Conversion3/1
  Demux/3 -> Data Type Conversion2/1
  Demux/6 -> Data Type Conversion5/1
  Demux/5 -> Data Type Conversion4/1
  Demux/8 -> Data Type Conversion7/1
  Demux/7 -> Data Type Conversion6/1
  Demux/10 -> Data Type Conversion9/1
  Demux/11 -> Data Type Conversion10/1
  Demux/12 -> Data Type Conversion11/1
  Demux/9 -> Data Type Conversion8/1
  Demux/13 -> Data Type Conversion12/1
  Demux/16 -> Data Type Conversion15/1
  Demux/14 -> Data Type Conversion13/1
  Demux/15 -> Data Type Conversion14/1
  Word to Bits/1 -> Demux/1
  Data Type Conversion/1 -> DATAOUT0/1
  Data Type Conversion1/1 -> DATAOUT1/1
  Data Type Conversion2/1 -> DATAOUT2/1
  Data Type Conversion3/1 -> DATAOUT3/1
  Data Type Conversion4/1 -> DATAOUT4/1
  Data Type Conversion5/1 -> DATAOUT5/1
  Data Type Conversion6/1 -> DATAOUT6/1
  Data Type Conversion7/1 -> DATAOUT7/1
  Data Type Conversion8/1 -> DATAOUT8/1
  Data Type Conversion9/1 -> DATAOUT9/1
  Data Type Conversion10/1 -> DATAOUT10/1
  Data Type Conversion11/1 -> DATAOUT11/1
  Data Type Conversion12/1 -> DATAOUT12/1
  Data Type Conversion13/1 -> DATAOUT13/1
  Data Type Conversion14/1 -> DATAOUT14/1
  Data Type Conversion15/1 -> DATAOUT15/1
  DATAIN/1 -> Word to Bits/1

== system UZ_EnDat_be4_optimizing_ctrs/UZ_ENDAT/Subsystem2/ManualDeserializere/ramwatcher ==
  In1 : Inport  OutMin=0  OutMax=32000  OutDataTypeStr=uint16  LockScale=on
  reset : Inport  Port=2  OutMin=0  OutMax=1  OutDataTypeStr=boolean  LockScale=on
  Trigger : TriggerPort  VariantControl=(inherit)  OutputDataType=int8  InitialTriggerSignalState=zero
  Constant2 : Constant  Value=0  OutDataTypeStr=uint16  SampleTime=-1
  Increment Stored Integer : hdlsllib/Math Operations/Increment Stored Integer
  Index Vector1 : MultiPortSwitch  DataPortOrder=Zero-based contiguous  Inputs=2  zeroidx=on  SaturateOnIntegerOverflow=off  InputSameDT=off
  SEL : Outport  InitialOutput=0
  wires:
  In1/1 -> Increment Stored Integer/1
  Increment Stored Integer/1 -> Index Vector1/2
  Index Vector1/1 -> SEL/1
  Constant2/1 -> Index Vector1/3
  reset/1 -> Index Vector1/1

== system UZ_EnDat_be4_optimizing_ctrs/UZ_ENDAT/responseslicer5/ENDAT23BITREVERSER/32BITREVERSE ==
  in : Inport
  16BITREVERSER : Subsystem
  16BITREVERSER1 : Subsystem
  Bit Concat : hdlsllib/Logic and Bit Operations/Bit Concat  numInputs=2
  Bit Slice : hdlsllib/Logic and Bit Operations/Bit Slice  lidx=15  ridx=0
  Bit Slice1 : hdlsllib/Logic and Bit Operations/Bit Slice  lidx=31  ridx=16
  out : Outport
  wires:
  in/1 -> Bit Slice1/1, Bit Slice/1
  16BITREVERSER/1(out) -> Bit Concat/1
  16BITREVERSER1/1(out) -> Bit Concat/2
  Bit Concat/1 -> out/1
  Bit Slice/1 -> 16BITREVERSER/1(in)
  Bit Slice1/1 -> 16BITREVERSER1/1(in)

== system UZ_EnDat_be4_optimizing_ctrs/UZ_ENDAT/timingprovider/CLKCNTER_POSCNTR/Positional_Counter ==
  valueout : Inport  OutDataTypeStr=uint32
  Trigger : TriggerPort  VariantControl=(inherit)  InitialTriggerSignalState=zero
  Increment Stored Integer : hdlsllib/Math Operations/Increment Stored Integer
  divider : Outport  InitialOutput=0
  wires:
  valueout/1 -> Increment Stored Integer/1
  Increment Stored Integer/1 -> divider/1

== system UZ_EnDat_be4_optimizing_ctrs/UZ_ENDAT/timingprovider/CLKCNTER_POSCNTR/SetZero32 ==
  valin : Inport
  setzero : Inport  Port=2  OutDataTypeStr=boolean
  Trigger : TriggerPort  TriggerType=either  VariantControl=(inherit)
  Constant1 : Constant  OutDataTypeStr=fixdt(0,1,0)  SampleTime=-1
  Constant2 : Constant  Value=0  OutDataTypeStr=fixdt(0,1,0)  SampleTime=-1
  Index Vector1 : MultiPortSwitch  DataPortOrder=Zero-based contiguous  Inputs=2  zeroidx=on  SaturateOnIntegerOverflow=off  InputSameDT=off
  Product : Product  OutDataTypeStr=uint32  RndMeth=Simplest  SaturateOnIntegerOverflow=on  LockScale=on
  valueout : Outport  InitialOutput=1  VectorParamsAs1DForOutWhenUnconnected=off
  wires:
  Index Vector1/1 -> Product/1
  valin/1 -> Product/2
  Product/1 -> valueout/1
  Constant1/1 -> Index Vector1/2
  Constant2/1 -> Index Vector1/3
  setzero/1 -> Index Vector1/1

== system UZ_EnDat_be4_optimizing_ctrs/UZ_ENDAT/timingprovider/CLKCNTER_POSCNTR/SetZero32modified ==
  valin : Inport
  setzero : Inport  Port=2  OutDataTypeStr=boolean
  Trigger : TriggerPort  TriggerType=either  VariantControl=(inherit)
  Constant2 : Constant  Value=0  OutDataTypeStr=uint32  SampleTime=-1
  Index Vector1 : MultiPortSwitch  DataPortOrder=Zero-based contiguous  Inputs=2  zeroidx=on  RndMeth=Simplest  InputSameDT=off
  valueout : Outport  InitialOutput=1  VectorParamsAs1DForOutWhenUnconnected=off
  wires:
  valin/1 -> Index Vector1/2
  Index Vector1/1 -> valueout/1
  Constant2/1 -> Index Vector1/3
  setzero/1 -> Index Vector1/1

== system UZ_EnDat_be4_optimizing_ctrs/UZ_ENDAT/timingprovider/CLKCNTER_POSCNTR/SetZero32modified1 ==
  valin : Inport
  setzero : Inport  Port=2  OutDataTypeStr=boolean
  Trigger : TriggerPort  TriggerType=either  VariantControl=(inherit)
  Constant2 : Constant  Value=0  OutDataTypeStr=uint32  SampleTime=-1
  Index Vector1 : MultiPortSwitch  DataPortOrder=Zero-based contiguous  Inputs=2  zeroidx=on  RndMeth=Simplest  InputSameDT=off
  valueout : Outport  InitialOutput=1  VectorParamsAs1DForOutWhenUnconnected=off
  wires:
  valin/1 -> Index Vector1/2
  Index Vector1/1 -> valueout/1
  Constant2/1 -> Index Vector1/3
  setzero/1 -> Index Vector1/1

== system UZ_EnDat_be4_optimizing_ctrs/UZ_ENDAT/timingprovider/CLKCNTER_POSCNTR1/Positional_Counter ==
  valueout : Inport  OutDataTypeStr=uint32
  Trigger : TriggerPort  VariantControl=(inherit)  InitialTriggerSignalState=zero
  Increment Stored Integer : hdlsllib/Math Operations/Increment Stored Integer
  divider : Outport  InitialOutput=0
  wires:
  valueout/1 -> Increment Stored Integer/1
  Increment Stored Integer/1 -> divider/1
